simulink model "mars_rover_ex_1a"  (R2023a)
settings: Solver=ode23t  StartTime=1  StopTime=abs(cam_pan_ex1(2)-cam_pan_ex1(1))/1  FixedStep=1e-2  MaxStep=0.05  RelTol=1e-3  AbsTol=1e-3  EnableMultiTasking=on
StartFcn:
  | mars_rover_ex1a_sim_callback
model workspace (MATLAB code in the model file):
  | addpath("mars_rover_helpers");
  | % Load Rover Arm model for IK
  | mdlpath = ['mars_rover_data',filesep,'mars_rover_arm'];
  | load_system(mdlpath);
  | 
  | imdata = zeros(3,3,3);
  | 
  | % Temp
  | Kp_steer = 1;
  | Ki_steer = 1;
  | Kd_steer = 1;
  | 
  | Kp = 1;
  | Ki = 1;
  | Kd = 1;
values from neighbouring files (symbols this model uses):
  cam_base_angle = 0    [mars_rover_params.m]
  cam_target_angle = 20    [mars_rover_params.m]
  mapData = false(197,200)    [mars_rover_params.m]    (also in mars_rover_startup.m)
  roverPath = app.rover_path    [NavigateOnMars.m]    (also in mars_rover_params.m = rover_path1)
undefined symbols (not defined in the file or in its folder): Arm, armJointAng, armJointTrqs, cam_pan_ex1, cam_pitch_ex1, cameraData, eeConfig, pose, Rover, sampleLocation, steerAng, steerTrqs, Terrain, vSpeed, Wheel1_G, Wheel2_G, Wheel3_G, Wheel4_G, Wheel5_G, Wheel6_G, wheelTrqs, wSpeeds, X, Y, Z
libraries: sm_lib x238, nesl_utility x80, slpidlib x3, simulink x3, robotcorelib x2, simulink_extras x2, robotalgslib x1
(part 2 of 9)

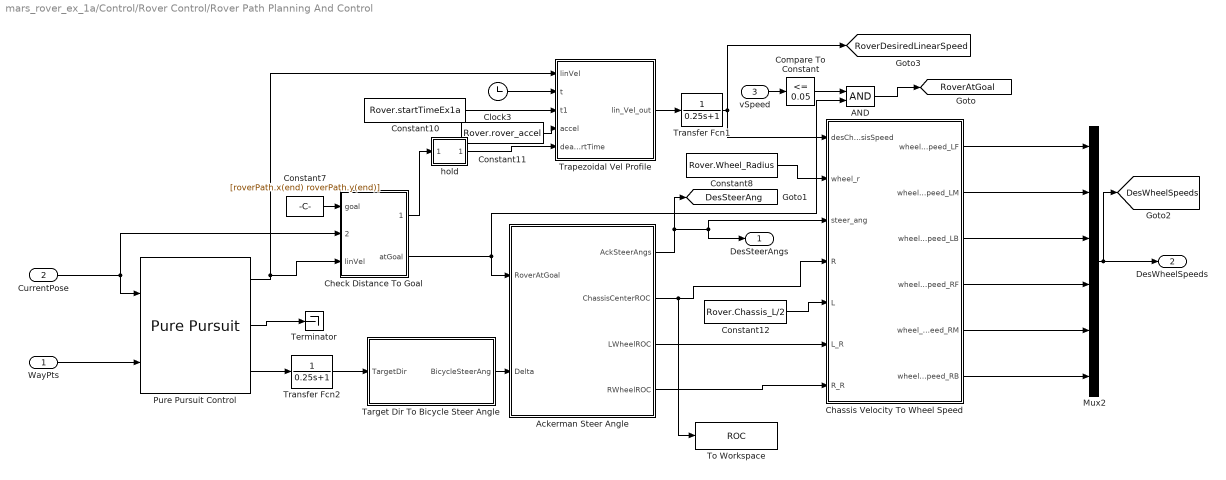
== system mars_rover_ex_1a/Control/Rover Control/Rover Path Planning And Control ==
  WayPts : Inport
  CurrentPose : Inport  Port=2
  vSpeed : Inport  Port=3
  AND : Logic  IconShape=distinctive  AllPortsSameDT=off  OutDataTypeStr=boolean
  Ackerman Steer Angle : Subsystem
  Chassis Velocity To Wheel Speed : MATLAB Function  TreatAsAtomicUnit=on
  Check Distance To Goal : Subsystem
  Clock3 : Clock
  Compare To Constant : simulink/Logic and Bit Operations/Compare To Constant  relop=<=  const=0.05  OutDataTypeStr=boolean
  Constant10 : Constant  Value=Rover.startTimeEx1a
  Constant11 : Constant  Value=Rover.rover_accel
  Constant12 : Constant  Value=Rover.Chassis_L/2
  Constant7 : Constant  Value=[roverPath.x(end) roverPath.y(end)]
  Constant8 : Constant  Value=Rover.Wheel_Radius
  Mux2 : Mux  Inputs=6
  Pure Pursuit Control : robotalgslib/Pure Pursuit  DesiredLinearVelocity=0.03  MaxAngularVelocity=0.01  LookaheadDistance=0.75  TargetDirPort=on  SimulateUsing=Code generation
  Target Dir To Bicycle Steer Angle : Subsystem  mask{L=Rover.Chassis_L/2, ld=0.75}
      mask prompts: L "Bicycle length"; ld "Lookahead distance"
      mask TypeOptions L: Bicycle length/Value
      mask TypeOptions ld: Lookahead distance/Value
  Terminator : Terminator
  To Workspace : ToWorkspace  VariableName=ROC  SampleTime=-1
  Transfer Fcn1 : TransferFcn  Denominator=[0.25 1]
  Transfer Fcn2 : TransferFcn  Denominator=[0.25 1]
  Trapezoidal Vel Profile : MATLAB Function  TreatAsAtomicUnit=on
  hold : Subsystem
  DesSteerAngs : Outport
  DesWheelSpeeds : Outport  Port=2
  tag scope: DesSteerAng=global, DesWheelSpeeds=global, RoverAtGoal=global, RoverDesiredLinearSpeed=global
  wires:
  Constant7/1 -> Check Distance To Goal/1(goal)
  CurrentPose/1 -> Pure Pursuit Control/1, Check Distance To Goal/2(currentPose)
  Check Distance To Goal/2(atGoal) -> Ackerman Steer Angle/1(RoverAtGoal), AND/2
  Clock3/1 -> Trapezoidal Vel Profile/2(t)
  Constant10/1 -> Trapezoidal Vel Profile/3(t1)
  Constant11/1 -> Trapezoidal Vel Profile/4(accel)
  Constant8/1 -> Chassis Velocity To Wheel Speed/2(wheel_r)
  Constant12/1 -> Chassis Velocity To Wheel Speed/5(L)
  Mux2/1 -> [DesWheelSpeeds], DesWheelSpeeds/1
  Check Distance To Goal/1(deAccel) -> hold/1(In1)
  hold/1(Out1) -> Trapezoidal Vel Profile/5(deaccelStartTime)
  Ackerman Steer Angle/1(AckSteerAngs) -> [DesSteerAng], Chassis Velocity To Wheel Speed/3(steer_ang), DesSteerAngs/1
  Target Dir To Bicycle Steer Angle/1(BicycleSteerAng) -> Ackerman Steer Angle/2(Delta)
  Ackerman Steer Angle/2(ChassisCenterROC) -> To Workspace/1, Chassis Velocity To Wheel Speed/4(R)
  Ackerman Steer Angle/3(LWheelROC) -> Chassis Velocity To Wheel Speed/6(L_R)
  Ackerman Steer Angle/4(RWheelROC) -> Chassis Velocity To Wheel Speed/7(R_R)
  Pure Pursuit Control/2 -> Terminator/1
  Compare To Constant/1 -> AND/1
  AND/1 -> [RoverAtGoal]
  Chassis Velocity To Wheel Speed/1(wheel_speed_LF) -> Mux2/1
  Chassis Velocity To Wheel Speed/2(wheel_speed_LM) -> Mux2/2
  Chassis Velocity To Wheel Speed/3(wheel_speed_LB) -> Mux2/3
  Chassis Velocity To Wheel Speed/4(wheel_speed_RF) -> Mux2/4
  Chassis Velocity To Wheel Speed/5(wheel_speed_RM) -> Mux2/5
  Chassis Velocity To Wheel Speed/6(wheel_speed_RB) -> Mux2/6
  Trapezoidal Vel Profile/1(lin_Vel_out) -> Transfer Fcn1/1
  vSpeed/1 -> Compare To Constant/1
  Transfer Fcn1/1 -> [RoverDesiredLinearSpeed], Chassis Velocity To Wheel Speed/1(desChassisSpeed)
  WayPts/1 -> Pure Pursuit Control/2
  Pure Pursuit Control/3 -> Transfer Fcn2/1
  Pure Pursuit Control/1 -> Trapezoidal Vel Profile/1(linVel), Check Distance To Goal/3(linVel)
  Transfer Fcn2/1 -> Target Dir To Bicycle Steer Angle/1(TargetDir)

== system mars_rover_ex_1a/Control/Rover Control/Steering Controller ==
  DesSteerAng : Inport
  ActSteerAng : Inport  Port=2
  Add : Sum  Inputs=+-
  Constant : Constant  Value=[Rover.Kp_steer,Rover.Ki_steer]
  Constant1 : Constant  Value=[10 1 ]
  Constant2 : Constant  Value=Rover.Kd_steer
  Constant3 : Constant  Value=Rover.N
  Demux : Demux  Outputs=2
  PID Controller1 : slpidlib/PID Controller  Controller=PID  Form=Parallel  TimeDomain=Continuous-time  UseExternalTs=off  SampleTime=-1  IntegratorMethod=Forward Euler  FilterMethod=Forward Euler  ControllerParametersSource=external  P=Kp_steer  I=Ki_steer  UseKiTs=off  D=Kd_steer  N=10  UseFilter=on  TunerSelectOption=Transfer Function Based (PID Tuner App)  InitialConditionSource=internal  InitialConditionForIntegrator=0  InitialConditionForFilter=0  DifferentiatorICPrevScaledInput=0  ExternalReset=none  TrackingMode=off  Kt=1  LimitOutput=off  SatLimitsSource=internal  UpperSaturationLimit=inf  LowerSaturationLimit=-inf  LinearizeAsGain=on  AntiWindupMode=none  Kb=1  POutMin=[]  POutMax=[]  IOutMin=[]  IOutMax=[]  DOutMin=[]  DOutMax=[]  NOutMin=[]  NOutMax=[]  SumOutMin=[]  SumOutMax=[]  SaturationOutMin=[]  SaturationOutMax=[]  PParamMin=[]  PParamMax=[]  IParamMin=[]  IParamMax=[]  DParamMin=[]  DParamMax=[]  NParamMin=[]  NParamMax=[]  KbParamMin=[]  KbParamMax=[]  KtParamMin=[]  KtParamMax=[]  KbOutMin=[]  KbOutMax=[]  KtOutMin=[]  KtOutMax=[]  IntegratorOutMin=[]  IntegratorOutMax=[]  FilterOutMin=[]  FilterOutMax=[]  SumI1OutMin=[]  SumI1OutMax=[]  SumI2OutMin=[]  SumI2OutMax=[]  SumI3OutMin=[]  SumI3OutMax=[]  SumI4OutMin=[]  SumI4OutMax=[]  SumDOutMin=[]  SumDOutMax=[]  DifferentiatorOutMin=[]  DifferentiatorOutMax=[]  FilterDiffOutCoefMin=[]  FilterDiffOutCoefMax=[]  ReciprocalOutMin=[]  ReciprocalOutMax=[]  SumDenOutMin=[]  SumDenOutMax=[]  SumNumOutMin=[]  SumNumOutMax=[]  DivideOutMin=[]  DivideOutMax=[]  UdiffTsProdOutMin=[]  UdiffTsProdOutMax=[]  NTsProdOutMin=[]  NTsProdOutMax=[]  UintegralTsProdOutMin=[]  UintegralTsProdOutMax=[]  UngainTsProdOutMin=[]  UngainTsProdOutMax=[]  IntegratorContinuousStateAttributes=''  IntegratorStateMustResolveToSignalObject=off  IntegratorRTWStateStorageClass=Auto  FilterContinuousStateAttributes=''  FilterStateMustResolveToSignalObject=off  FilterRTWStateStorageClass=Auto  ParallelPVariant=ExternalParameters  IdealPVariant=Disabled  IVariant=ExternalParameters  DVariant=ExternalParameters  IntegratorVariant=Continuous  SatVariant=Disabled  AWVariant=Passthrough  PCopyVariant=Disabled  TRVariant=Disabled  FdbkBlocksVariant=Forward  IdealPFdbkVariant=Disabled  SatFdbkVariant=Disabled  DerivativeFilterVariant=ContFilter  NVariant=ExternalParameters  NCopyVariant=Disabled  FilterICVariant=InternalICsFilter  IntegratorICVariant=InternalICs  ExternalResetVariant=Disabled  TRSumVariant=Passthrough  SumFdbkVariant=Disabled  SumVariant=Sum_PID  TsampFilterVariant=InternalTs  TsampNgainVariant=Passthrough  TsampIntegralVariant=Passthrough  ExternalSaturationOutDataTypeStr=Inherit: Same as second input
  Subsystem : Subsystem  mask(First-order lag supporting vector signals){b=[1 1 1 1]*0.05, x_initial=[0 0 0 0]}
      mask prompts: b "Filter time constant"; x_initial "Initial output"
      mask help: Models a lag of the form 1/(b*s+1) where s is the Laplace operator.
  Subsystem1 : Subsystem  mask(First-order lag supporting vector signals){b=[1 1 1 1]*0.05, x_initial=[0 0 0 0]}
      mask prompts: b "Filter time constant"; x_initial "Initial output"
      mask help: Models a lag of the form 1/(b*s+1) where s is the Laplace operator.
  Switch : Switch  Criteria=u2 > Threshold  SaturateOnIntegerOverflow=off  InputSameDT=off
  SteerTrqs : Outport
  wires:
  PID Controller1/1 -> SteerTrqs/1
  Add/1 -> PID Controller1/1
  [RoverAtGoal] -> Switch/2
  Constant1/1 -> Switch/1
  Demux/1 -> PID Controller1/2
  Demux/2 -> PID Controller1/3
  Constant/1 -> Switch/3
  Switch/1 -> Demux/1
  DesSteerAng/1 -> Subsystem/1(In)
  ActSteerAng/1 -> Subsystem1/1(In)
  Subsystem/1(out) -> Add/1
  Subsystem1/1(out) -> Add/2
  Constant2/1 -> PID Controller1/4
  Constant3/1 -> PID Controller1/5

== system mars_rover_ex_1a/Control/Rover Control/Wheel Speed Controller ==
  DesWheelSpeeds : Inport
  ActWheelSpeed : Inport  Port=2
  Add3 : Sum  Inputs=+-
  Constant : Constant  Value=[Rover.Kp,Rover.Ki]
  Constant1 : Constant  Value=[5000 100 ]
  Constant2 : Constant  Value=Rover.Kd
  Constant3 : Constant  Value=Rover.N
  Demux : Demux  Outputs=2
  PID Controller3 : slpidlib/PID Controller  Controller=PID  Form=Parallel  TimeDomain=Continuous-time  UseExternalTs=off  SampleTime=-1  IntegratorMethod=Forward Euler  FilterMethod=Forward Euler  ControllerParametersSource=external  P=Kp  I=Ki  UseKiTs=off  D=Kd  N=100  UseFilter=on  TunerSelectOption=Transfer Function Based (PID Tuner App)  InitialConditionSource=internal  InitialConditionForIntegrator=0  InitialConditionForFilter=0  DifferentiatorICPrevScaledInput=0  ExternalReset=none  TrackingMode=off  Kt=1  LimitOutput=off  SatLimitsSource=internal  UpperSaturationLimit=inf  LowerSaturationLimit=-inf  LinearizeAsGain=on  AntiWindupMode=none  Kb=1  POutMin=[]  POutMax=[]  IOutMin=[]  IOutMax=[]  DOutMin=[]  DOutMax=[]  NOutMin=[]  NOutMax=[]  SumOutMin=[]  SumOutMax=[]  SaturationOutMin=[]  SaturationOutMax=[]  PParamMin=[]  PParamMax=[]  IParamMin=[]  IParamMax=[]  DParamMin=[]  DParamMax=[]  NParamMin=[]  NParamMax=[]  KbParamMin=[]  KbParamMax=[]  KtParamMin=[]  KtParamMax=[]  KbOutMin=[]  KbOutMax=[]  KtOutMin=[]  KtOutMax=[]  IntegratorOutMin=[]  IntegratorOutMax=[]  FilterOutMin=[]  FilterOutMax=[]  SumI1OutMin=[]  SumI1OutMax=[]  SumI2OutMin=[]  SumI2OutMax=[]  SumI3OutMin=[]  SumI3OutMax=[]  SumI4OutMin=[]  SumI4OutMax=[]  SumDOutMin=[]  SumDOutMax=[]  DifferentiatorOutMin=[]  DifferentiatorOutMax=[]  FilterDiffOutCoefMin=[]  FilterDiffOutCoefMax=[]  ReciprocalOutMin=[]  ReciprocalOutMax=[]  SumDenOutMin=[]  SumDenOutMax=[]  SumNumOutMin=[]  SumNumOutMax=[]  DivideOutMin=[]  DivideOutMax=[]  UdiffTsProdOutMin=[]  UdiffTsProdOutMax=[]  NTsProdOutMin=[]  NTsProdOutMax=[]  UintegralTsProdOutMin=[]  UintegralTsProdOutMax=[]  UngainTsProdOutMin=[]  UngainTsProdOutMax=[]  IntegratorContinuousStateAttributes=''  IntegratorStateMustResolveToSignalObject=off  IntegratorRTWStateStorageClass=Auto  FilterContinuousStateAttributes=''  FilterStateMustResolveToSignalObject=off  FilterRTWStateStorageClass=Auto  ParallelPVariant=ExternalParameters  IdealPVariant=Disabled  IVariant=ExternalParameters  DVariant=ExternalParameters  IntegratorVariant=Continuous  SatVariant=Disabled  AWVariant=Passthrough  PCopyVariant=Disabled  TRVariant=Disabled  FdbkBlocksVariant=Forward  IdealPFdbkVariant=Disabled  SatFdbkVariant=Disabled  DerivativeFilterVariant=ContFilter  NVariant=ExternalParameters  NCopyVariant=Disabled  FilterICVariant=InternalICsFilter  IntegratorICVariant=InternalICs  ExternalResetVariant=Disabled  TRSumVariant=Passthrough  SumFdbkVariant=Disabled  SumVariant=Sum_PID  TsampFilterVariant=InternalTs  TsampNgainVariant=Passthrough  TsampIntegralVariant=Passthrough  ExternalSaturationOutDataTypeStr=Inherit: Same as second input
  Saturation : Saturate  UpperLimit=Rover.TrqUpLimit  LowerLimit=Rover.TrqLoLimit
  Subsystem : Subsystem  mask(First-order lag supporting vector signals){b=[1 1 1 1 1 1]*0.05, x_initial=[0 0 0 0 0 0]}
      mask prompts: b "Filter time constant"; x_initial "Initial output"
      mask help: Models a lag of the form 1/(b*s+1) where s is the Laplace operator.
  Subsystem1 : Subsystem  mask(First-order lag supporting vector signals){b=[1 1 1 1 1 1]*0.05, x_initial=[0 0 0 0 0 0]}
      mask prompts: b "Filter time constant"; x_initial "Initial output"
      mask help: Models a lag of the form 1/(b*s+1) where s is the Laplace operator.
  Switch : Switch  Criteria=u2 > Threshold  SaturateOnIntegerOverflow=off  InputSameDT=off
  WheelTrqs : Outport
  wires:
  Saturation/1 -> WheelTrqs/1
  Switch/1 -> Demux/1
  Constant/1 -> Switch/3
  Constant1/1 -> Switch/1
  Demux/2 -> PID Controller3/3
  Demux/1 -> PID Controller3/2
  [RoverAtGoal] -> Switch/2
  PID Controller3/1 -> Saturation/1
  Add3/1 -> PID Controller3/1
  DesWheelSpeeds/1 -> Subsystem/1(In)
  ActWheelSpeed/1 -> Subsystem1/1(In)
  Subsystem/1(out) -> Add3/1
  Subsystem1/1(out) -> Add3/2
  Constant3/1 -> PID Controller3/5
  Constant2/1 -> PID Controller3/4

== system mars_rover_ex_1a/Mars Rover Plant/Manipulator Plant Model/End Effector Sense ==
  Mux1 : Mux  Inputs=3
  PS-Simulink Converter6 : nesl_utility/PS-Simulink Converter  PhysicalDomain=network_engine_domain  SubClassName=ps_output  LeftPortType=input  RightPortType=output  PseudoPeriodic=off  Frequencies=[]  VectorFormat=1-D array  Unit=inherit  AffineConversion=off
  PS-Simulink Converter7 : nesl_utility/PS-Simulink Converter  PhysicalDomain=network_engine_domain  SubClassName=ps_output  LeftPortType=input  RightPortType=output  PseudoPeriodic=off  Frequencies=[]  VectorFormat=1-D array  Unit=inherit  AffineConversion=off
  PS-Simulink Converter8 : nesl_utility/PS-Simulink Converter  PhysicalDomain=network_engine_domain  SubClassName=ps_output  LeftPortType=input  RightPortType=output  PseudoPeriodic=off  Frequencies=[]  VectorFormat=1-D array  Unit=inherit  AffineConversion=off
  Terminator : Terminator
  Transform Sensor : sm_lib/Frames and Transforms/Transform Sensor  MeasurementFrame=Base  RotationSequence=XYX  SenseAngle=off  SenseAxis=off  SenseQ=off  SenseR=off  SenseRotationSequence=off  SenseOmegaX=off  SenseOmegaY=off  SenseOmegaZ=off  SenseQDot=off  SenseRDot=off  SenseRotationSequenceDot=off  SenseAlphaX=off  SenseAlphaY=off  SenseAlphaZ=off  SenseQDDot=off  SenseRDDot=off  SenseX=on  SenseY=on  SenseZ=on  SenseRad=off  SenseAzim=off  SenseDist=off  SenseInc=off  SenseXDot=off  SenseYDot=off  SenseZDot=off  SenseRadDot=off  SenseAzimDot=off  SenseDistDot=off  SenseIncDot=off  SenseXDDot=off  SenseYDDot=off  SenseZDDot=off  SenseRadDDot=off  SenseAzimDDot=off  SenseDistDDot=off  SenseIncDDot=off
  ArmB : PMIOPort  Side=Left
  EndEff : PMIOPort  Port=2  Side=Right
  wires:
  PS-Simulink Converter8/1 -> Mux1/3
  PS-Simulink Converter7/1 -> Mux1/2
  PS-Simulink Converter6/1 -> Mux1/1
  Mux1/1 -> Terminator/1  "endEffPos"
  connections:
  Transform Sensor/RConn1 -- EndEff/RConn1
  PS-Simulink Converter8/LConn1 -- Transform Sensor/RConn4
  PS-Simulink Converter7/LConn1 -- Transform Sensor/RConn3
  PS-Simulink Converter6/LConn1 -- Transform Sensor/RConn2
  ArmB/RConn1 -- Transform Sensor/LConn1

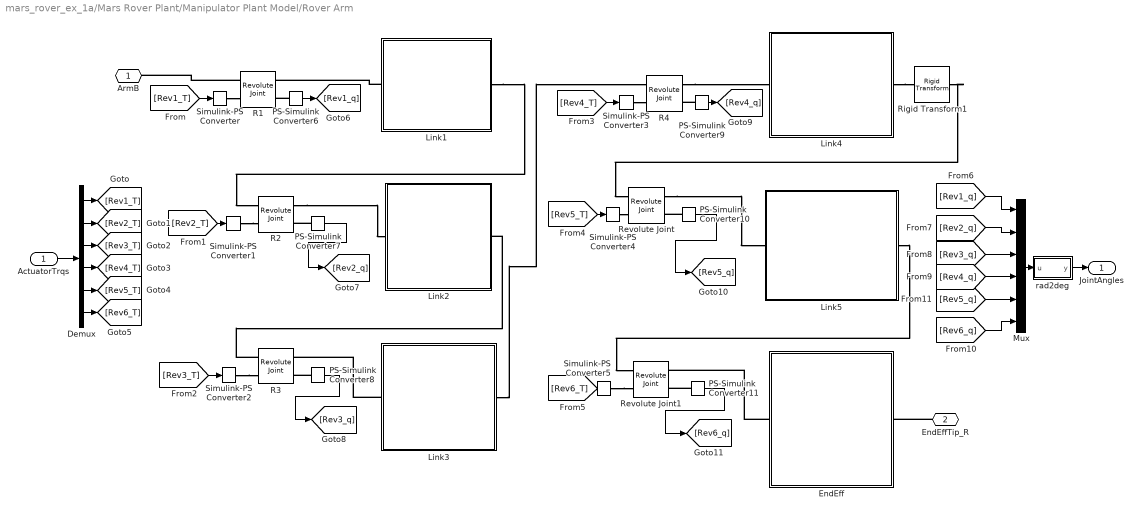
== system mars_rover_ex_1a/Mars Rover Plant/Manipulator Plant Model/Rover Arm ==
  ActuatorTrqs : Inport
  Demux : Demux  Outputs=6
  EndEff : Subsystem
      mask Display: image('$imagefile'); % Use "Edit Image" on toolstrip to change.
  Link1 : Subsystem
      mask Display: image('$imagefile'); % Use "Edit Image" on toolstrip to change.
  Link2 : Subsystem
      mask Display: image('$imagefile'); % Use "Edit Image" on toolstrip to change.
  Link3 : Subsystem
      mask Display: image('$imagefile'); % Use "Edit Image" on toolstrip to change.
  Link4 : Subsystem
      mask Display: image('$imagefile'); % Use "Edit Image" on toolstrip to change.
  Link5 : Subsystem
      mask Display: image('$imagefile'); % Use "Edit Image" on toolstrip to change.
  Mux : Mux  Inputs=6
  PS-Simulink Converter{6..11} (6 alike) : nesl_utility/PS-Simulink Converter  PhysicalDomain=network_engine_domain  SubClassName=ps_output  LeftPortType=input  RightPortType=output  PseudoPeriodic=off  Frequencies=[]  VectorFormat=1-D array  Unit=inherit  AffineConversion=off
  R1 : sm_lib/Joints/Revolute Joint  JointMode=Normal  SenseConstraintForce=off  SenseConstraintForceX=off  SenseConstraintForceY=off  SenseConstraintForceZ=off  SenseConstraintTorque=off  SenseConstraintTorqueX=off  SenseConstraintTorqueY=off  SenseConstraintTorqueZ=off  SenseTotalForce=off  SenseTotalForceX=off  SenseTotalForceY=off  SenseTotalForceZ=off  SenseTotalTorque=off  SenseTotalTorqueX=off  SenseTotalTorqueY=off  SenseTotalTorqueZ=off  CompositeWrenchDir=FollowerOnBase  CompositeWrenchFrame=BaseFrame  EquilibriumPosition=0  EquilibriumPositionUnits=deg  SpringStiffness=0  SpringStiffnessUnits=N*m/deg  DampingCoefficient=Arm.D  DampingCoefficientUnits=N*m/(deg/s)  TorqueActuationMode=InputTorque  MotionActuationMode=ComputedMotion  SensePosition=on  SenseVelocity=off  SenseAcceleration=off  SenseTorqueForce=off  SenseLowerLimitTorqueForce=off  SenseUpperLimitTorqueForce=off  LowerLimitSpecify=off  LowerLimitBound=-90  LowerLimitBoundUnits=deg  LowerLimitStiffness=1e4  LowerLimitStiffnessUnits=N*m/deg  LowerLimitDamping=10  LowerLimitDampingUnits=N*m/(deg/s)  LowerLimitTransitionRegionWidth=0.1  LowerLimitTransitionRegionWidthUnits=deg  UpperLimitSpecify=off  UpperLimitBound=90  UpperLimitBoundUnits=deg  UpperLimitStiffness=1e4  UpperLimitStiffnessUnits=N*m/deg  UpperLimitDamping=10  UpperLimitDampingUnits=N*m/(deg/s)  UpperLimitTransitionRegionWidth=0.1  UpperLimitTransitionRegionWidthUnits=deg  PositionTargetSpecify=on  PositionTargetPriority=High  PositionTargetValue=Arm.arm_q0(1)  PositionTargetValueUnits=deg  VelocityTargetSpecify=off  VelocityTargetPriority=High  VelocityTargetValue=0  VelocityTargetValueUnits=deg/s
  R2 : sm_lib/Joints/Revolute Joint  JointMode=Normal  SenseConstraintForce=off  SenseConstraintForceX=off  SenseConstraintForceY=off  SenseConstraintForceZ=off  SenseConstraintTorque=off  SenseConstraintTorqueX=off  SenseConstraintTorqueY=off  SenseConstraintTorqueZ=off  SenseTotalForce=off  SenseTotalForceX=off  SenseTotalForceY=off  SenseTotalForceZ=off  SenseTotalTorque=off  SenseTotalTorqueX=off  SenseTotalTorqueY=off  SenseTotalTorqueZ=off  CompositeWrenchDir=FollowerOnBase  CompositeWrenchFrame=BaseFrame  EquilibriumPosition=0  EquilibriumPositionUnits=deg  SpringStiffness=0  SpringStiffnessUnits=N*m/deg  DampingCoefficient=Arm.D  DampingCoefficientUnits=N*m/(deg/s)  TorqueActuationMode=InputTorque  MotionActuationMode=ComputedMotion  SensePosition=on  SenseVelocity=off  SenseAcceleration=off  SenseTorqueForce=off  SenseLowerLimitTorqueForce=off  SenseUpperLimitTorqueForce=off  LowerLimitSpecify=off  LowerLimitBound=-90  LowerLimitBoundUnits=deg  LowerLimitStiffness=1e4  LowerLimitStiffnessUnits=N*m/deg  LowerLimitDamping=10  LowerLimitDampingUnits=N*m/(deg/s)  LowerLimitTransitionRegionWidth=0.1  LowerLimitTransitionRegionWidthUnits=deg  UpperLimitSpecify=off  UpperLimitBound=90  UpperLimitBoundUnits=deg  UpperLimitStiffness=1e4  UpperLimitStiffnessUnits=N*m/deg  UpperLimitDamping=10  UpperLimitDampingUnits=N*m/(deg/s)  UpperLimitTransitionRegionWidth=0.1  UpperLimitTransitionRegionWidthUnits=deg  PositionTargetSpecify=on  PositionTargetPriority=High  PositionTargetValue=Arm.arm_q0(2)  PositionTargetValueUnits=deg  VelocityTargetSpecify=off  VelocityTargetPriority=High  VelocityTargetValue=0  VelocityTargetValueUnits=deg/s
  R3 : sm_lib/Joints/Revolute Joint  JointMode=Normal  SenseConstraintForce=off  SenseConstraintForceX=off  SenseConstraintForceY=off  SenseConstraintForceZ=off  SenseConstraintTorque=off  SenseConstraintTorqueX=off  SenseConstraintTorqueY=off  SenseConstraintTorqueZ=off  SenseTotalForce=off  SenseTotalForceX=off  SenseTotalForceY=off  SenseTotalForceZ=off  SenseTotalTorque=off  SenseTotalTorqueX=off  SenseTotalTorqueY=off  SenseTotalTorqueZ=off  CompositeWrenchDir=FollowerOnBase  CompositeWrenchFrame=BaseFrame  EquilibriumPosition=0  EquilibriumPositionUnits=deg  SpringStiffness=0  SpringStiffnessUnits=N*m/deg  DampingCoefficient=Arm.D  DampingCoefficientUnits=N*m/(deg/s)  TorqueActuationMode=InputTorque  MotionActuationMode=ComputedMotion  SensePosition=on  SenseVelocity=off  SenseAcceleration=off  SenseTorqueForce=off  SenseLowerLimitTorqueForce=off  SenseUpperLimitTorqueForce=off  LowerLimitSpecify=off  LowerLimitBound=-10  LowerLimitBoundUnits=deg  LowerLimitStiffness=1e4  LowerLimitStiffnessUnits=N*m/deg  LowerLimitDamping=10  LowerLimitDampingUnits=N*m/(deg/s)  LowerLimitTransitionRegionWidth=0.1  LowerLimitTransitionRegionWidthUnits=deg  UpperLimitSpecify=off  UpperLimitBound=160  UpperLimitBoundUnits=deg  UpperLimitStiffness=1e4  UpperLimitStiffnessUnits=N*m/deg  UpperLimitDamping=10  UpperLimitDampingUnits=N*m/(deg/s)  UpperLimitTransitionRegionWidth=0.1  UpperLimitTransitionRegionWidthUnits=deg  PositionTargetSpecify=on  PositionTargetPriority=High  PositionTargetValue=Arm.arm_q0(3)  PositionTargetValueUnits=deg  VelocityTargetSpecify=off  VelocityTargetPriority=High  VelocityTargetValue=0  VelocityTargetValueUnits=deg/s
  R4 : sm_lib/Joints/Revolute Joint  JointMode=Normal  SenseConstraintForce=off  SenseConstraintForceX=off  SenseConstraintForceY=off  SenseConstraintForceZ=off  SenseConstraintTorque=off  SenseConstraintTorqueX=off  SenseConstraintTorqueY=off  SenseConstraintTorqueZ=off  SenseTotalForce=off  SenseTotalForceX=off  SenseTotalForceY=off  SenseTotalForceZ=off  SenseTotalTorque=off  SenseTotalTorqueX=off  SenseTotalTorqueY=off  SenseTotalTorqueZ=off  CompositeWrenchDir=FollowerOnBase  CompositeWrenchFrame=BaseFrame  EquilibriumPosition=0  EquilibriumPositionUnits=deg  SpringStiffness=0  SpringStiffnessUnits=N*m/deg  DampingCoefficient=Arm.D  DampingCoefficientUnits=N*m/(deg/s)  TorqueActuationMode=InputTorque  MotionActuationMode=ComputedMotion  SensePosition=on  SenseVelocity=off  SenseAcceleration=off  SenseTorqueForce=off  SenseLowerLimitTorqueForce=off  SenseUpperLimitTorqueForce=off  LowerLimitSpecify=off  LowerLimitBound=-90  LowerLimitBoundUnits=deg  LowerLimitStiffness=1e4  LowerLimitStiffnessUnits=N*m/deg  LowerLimitDamping=10  LowerLimitDampingUnits=N*m/(deg/s)  LowerLimitTransitionRegionWidth=0.1  LowerLimitTransitionRegionWidthUnits=deg  UpperLimitSpecify=off  UpperLimitBound=90  UpperLimitBoundUnits=deg  UpperLimitStiffness=1e4  UpperLimitStiffnessUnits=N*m/deg  UpperLimitDamping=10  UpperLimitDampingUnits=N*m/(deg/s)  UpperLimitTransitionRegionWidth=0.1  UpperLimitTransitionRegionWidthUnits=deg  PositionTargetSpecify=on  PositionTargetPriority=High  PositionTargetValue=Arm.arm_q0(4)  PositionTargetValueUnits=deg  VelocityTargetSpecify=off  VelocityTargetPriority=High  VelocityTargetValue=0  VelocityTargetValueUnits=deg/s
  Revolute Joint : sm_lib/Joints/Revolute Joint  JointMode=Normal  SenseConstraintForce=off  SenseConstraintForceX=off  SenseConstraintForceY=off  SenseConstraintForceZ=off  SenseConstraintTorque=off  SenseConstraintTorqueX=off  SenseConstraintTorqueY=off  SenseConstraintTorqueZ=off  SenseTotalForce=off  SenseTotalForceX=off  SenseTotalForceY=off  SenseTotalForceZ=off  SenseTotalTorque=off  SenseTotalTorqueX=off  SenseTotalTorqueY=off  SenseTotalTorqueZ=off  CompositeWrenchDir=FollowerOnBase  CompositeWrenchFrame=BaseFrame  EquilibriumPosition=0  EquilibriumPositionUnits=deg  SpringStiffness=0  SpringStiffnessUnits=N*m/deg  DampingCoefficient=Arm.D2  DampingCoefficientUnits=N*m/(deg/s)  TorqueActuationMode=InputTorque  MotionActuationMode=ComputedMotion  SensePosition=on  SenseVelocity=off  SenseAcceleration=off  SenseTorqueForce=off  SenseLowerLimitTorqueForce=off  SenseUpperLimitTorqueForce=off  LowerLimitSpecify=off  LowerLimitBound=-90  LowerLimitBoundUnits=deg  LowerLimitStiffness=1e4  LowerLimitStiffnessUnits=N*m/deg  LowerLimitDamping=10  LowerLimitDampingUnits=N*m/(deg/s)  LowerLimitTransitionRegionWidth=0.1  LowerLimitTransitionRegionWidthUnits=deg  UpperLimitSpecify=off  UpperLimitBound=90  UpperLimitBoundUnits=deg  UpperLimitStiffness=1e4  UpperLimitStiffnessUnits=N*m/deg  UpperLimitDamping=10  UpperLimitDampingUnits=N*m/(deg/s)  UpperLimitTransitionRegionWidth=0.1  UpperLimitTransitionRegionWidthUnits=deg  PositionTargetSpecify=on  PositionTargetPriority=High  PositionTargetValue=Arm.arm_q0(5)  PositionTargetValueUnits=deg  VelocityTargetSpecify=off  VelocityTargetPriority=High  VelocityTargetValue=0  VelocityTargetValueUnits=deg/s
  Revolute Joint1 : sm_lib/Joints/Revolute Joint  JointMode=Normal  SenseConstraintForce=off  SenseConstraintForceX=off  SenseConstraintForceY=off  SenseConstraintForceZ=off  SenseConstraintTorque=off  SenseConstraintTorqueX=off  SenseConstraintTorqueY=off  SenseConstraintTorqueZ=off  SenseTotalForce=off  SenseTotalForceX=off  SenseTotalForceY=off  SenseTotalForceZ=off  SenseTotalTorque=off  SenseTotalTorqueX=off  SenseTotalTorqueY=off  SenseTotalTorqueZ=off  CompositeWrenchDir=FollowerOnBase  CompositeWrenchFrame=BaseFrame  EquilibriumPosition=0  EquilibriumPositionUnits=deg  SpringStiffness=0  SpringStiffnessUnits=N*m/deg  DampingCoefficient=Arm.D2  DampingCoefficientUnits=N*m/(deg/s)  TorqueActuationMode=InputTorque  MotionActuationMode=ComputedMotion  SensePosition=on  SenseVelocity=off  SenseAcceleration=off  SenseTorqueForce=off  SenseLowerLimitTorqueForce=off  SenseUpperLimitTorqueForce=off  LowerLimitSpecify=off  LowerLimitBound=-90  LowerLimitBoundUnits=deg  LowerLimitStiffness=1e4  LowerLimitStiffnessUnits=N*m/deg  LowerLimitDamping=10  LowerLimitDampingUnits=N*m/(deg/s)  LowerLimitTransitionRegionWidth=0.1  LowerLimitTransitionRegionWidthUnits=deg  UpperLimitSpecify=off  UpperLimitBound=90  UpperLimitBoundUnits=deg  UpperLimitStiffness=1e4  UpperLimitStiffnessUnits=N*m/deg  UpperLimitDamping=10  UpperLimitDampingUnits=N*m/(deg/s)  UpperLimitTransitionRegionWidth=0.1  UpperLimitTransitionRegionWidthUnits=deg  PositionTargetSpecify=on  PositionTargetPriority=High  PositionTargetValue=Arm.arm_q0(6)  PositionTargetValueUnits=deg  VelocityTargetSpecify=off  VelocityTargetPriority=High  VelocityTargetValue=0  VelocityTargetValueUnits=deg/s
  Rigid Transform1 : sm_lib/Frames and Transforms/Rigid Transform  TranslationMethod=StandardAxis  TranslationStandardOffset=3  TranslationStandardOffsetUnits=cm  TranslationStandardAxis=+Z  TranslationCartesianOffset=[0 0 0]  TranslationCartesianOffsetUnits=cm  TranslationROffset=0  TranslationROffsetUnits=m  TranslationZOffset=0  TranslationZOffsetUnits=m  TranslationThetaOffset=0  TranslationThetaOffsetUnits=deg  RotationMethod=None  RotationAngleUnits=deg  RotationStandardAxis=+X  RotationAngle=90  RotationArbitraryAxis=[0 0 1]  FollAlignAxisA=+X  BaseAlignAxisA=+Y  FollAlignAxisB=+Y  BaseAlignAxisB=+Z  RotationSequenceAxes=FollowerAxes  RotationSequence=XYX  RotationSequenceAngles=[0 0 0]  RotationSequenceAnglesUnits=deg  RotationMatrix=[1 0 0; 0 1 0; 0 0 1]  Quaternion=[1 0 0 0]
  Simulink-PS Converter{,1..5} (6 alike) : nesl_utility/Simulink-PS Converter  PhysicalDomain=network_engine_domain  SubClassName=ps_input  LeftPortType=input  RightPortType=output  PseudoPeriodic=off  Frequencies=[]  NoiseDistribution=none  NoiseParameters=[]  Unit=1  AffineConversion=off  FilteringAndDerivatives=provide  SimscapeFilterOrder=1  InputFilterTimeConstant=0.001  UdotUserProvided=0
  rad2deg : MATLAB Function  TreatAsAtomicUnit=on
  ArmB : PMIOPort  Side=Left
  EndEffTip_R : PMIOPort  Port=2  Side=Right
  JointAngles : Outport
  wires:
  Mux/1 -> rad2deg/1(u)
  [Rev2_q] -> Mux/2
  [Rev3_q] -> Mux/3
  [Rev4_q] -> Mux/4
  [Rev5_q] -> Mux/5
  [Rev6_q] -> Mux/6
  ActuatorTrqs/1 -> Demux/1
  Demux/1 -> [Rev1_T]
  Demux/2 -> [Rev2_T]
  Demux/3 -> [Rev3_T]
  Demux/4 -> [Rev4_T]
  Demux/5 -> [Rev5_T]
  Demux/6 -> [Rev6_T]
  [Rev1_T] -> Simulink-PS Converter/1
  [Rev2_T] -> Simulink-PS Converter1/1
  [Rev3_T] -> Simulink-PS Converter2/1
  [Rev4_T] -> Simulink-PS Converter3/1
  [Rev5_T] -> Simulink-PS Converter4/1
  [Rev6_T] -> Simulink-PS Converter5/1
  PS-Simulink Converter6/1 -> [Rev1_q]
  PS-Simulink Converter7/1 -> [Rev2_q]
  PS-Simulink Converter8/1 -> [Rev3_q]
  PS-Simulink Converter9/1 -> [Rev4_q]
  PS-Simulink Converter10/1 -> [Rev5_q]
  PS-Simulink Converter11/1 -> [Rev6_q]
  rad2deg/1(y) -> JointAngles/1
  [Rev1_q] -> Mux/1
  connections:
  Link1/LConn1 -- R1/RConn1
  Link3/RConn1 -- R4/LConn1
  R2/RConn1 -- Link2/LConn1
  R3/LConn1 -- Link2/RConn1
  R4/RConn1 -- Link4/LConn1
  Link1/RConn1 -- R2/LConn1
  Link3/LConn1 -- R3/RConn1
  Link4/RConn1 -- Rigid Transform1/LConn1
  EndEff/LConn1 -- Revolute Joint1/RConn1
  Rigid Transform1/RConn1 -- Revolute Joint/LConn1
  EndEffTip_R/RConn1 -- EndEff/RConn1
  R1/LConn1 -- ArmB/RConn1
  Link5/RConn1 -- Revolute Joint1/LConn1
  Revolute Joint/RConn1 -- Link5/LConn1
  Simulink-PS Converter/RConn1 -- R1/LConn2
  Simulink-PS Converter1/RConn1 -- R2/LConn2
  Simulink-PS Converter2/RConn1 -- R3/LConn2
  Simulink-PS Converter3/RConn1 -- R4/LConn2
  Simulink-PS Converter4/RConn1 -- Revolute Joint/LConn2
  Simulink-PS Converter5/RConn1 -- Revolute Joint1/LConn2
  PS-Simulink Converter6/LConn1 -- R1/RConn2
  PS-Simulink Converter7/LConn1 -- R2/RConn2
  PS-Simulink Converter8/LConn1 -- R3/RConn2
  PS-Simulink Converter9/LConn1 -- R4/RConn2
  PS-Simulink Converter10/LConn1 -- Revolute Joint/RConn2
  PS-Simulink Converter11/LConn1 -- Revolute Joint1/RConn2
